simulink library "halin"  (R2021b)
settings: Solver=VariableStepAuto  StartTime=0.0  StopTime=10.0  RelTol=1e-3
undefined symbols (not defined in the file): TRUE
libraries: FVT_lib x177, hcu_lib x55
(part 6 of 17)

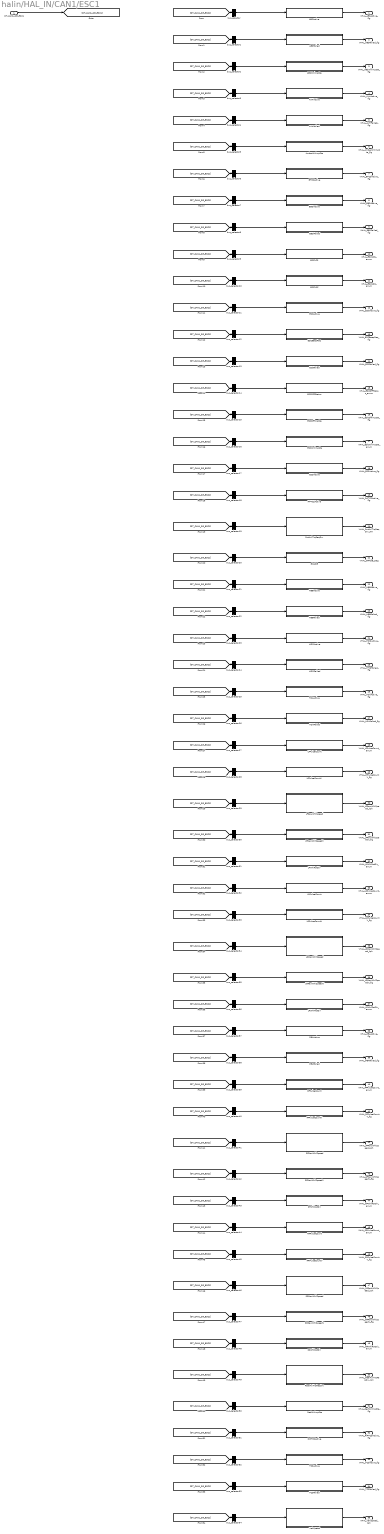
== system halin/HAL_IN/CAN1/ESC1 ==
  DT_CAN1_SG_ESC1 : Inport
  ABSActive : Subsystem
  ABSFailed : Subsystem
  ABSWnlmpSta : Subsystem
  AVHActive : Subsystem
  AVHFailed : Subsystem
  AmberWnlmpSta : Subsystem
  BTCSActive : Subsystem
  EBDActive : Subsystem
  EBDFailed : Subsystem
  ESC1CS : Subsystem
  ESC1RC : Subsystem
  ESCActive : Subsystem
  ESCBeepReq : Subsystem
  ESCFailed : Subsystem
  ESCOFFStatus : Subsystem
  ESCOfflmpSta : Subsystem
  ESCWnlmpSta : Subsystem
  ESSActive : Subsystem
  FrPTCSActive : Subsystem
  FrntAxlTrqReqDrv : Subsystem
  GRADE : Subsystem
  HBBActive : Subsystem
  HBBFailed : Subsystem
  HDDActive : Subsystem
  HDDFailed : Subsystem
  HSAActive : Subsystem
  HSAFailed : Subsystem
  LFPulseCount : Subsystem
  LFPulseCountV : Subsystem
  LFRawWhlSpeed : Subsystem
  LFRawWhlSpeedV : Subsystem
  LFWhlRotDir : Subsystem
  LRPulseCount : Subsystem
  LRPulseCountV : Subsystem
  LRRawWhlSpeed : Subsystem
  LRRawWhlSpeedV : Subsystem
  LRWhlRotDir : Subsystem
  PBAActive : Subsystem
  PBAFailed : Subsystem
  RFPulseCount : Subsystem
  RFPulseCountV : Subsystem
  RFRawWhlSpeed : Subsystem
  RFRawWhlSpeedV : Subsystem
  RFWhlRotDir : Subsystem
  RRPulseCount : Subsystem
  RRPulseCountV : Subsystem
  RRRawWhlSpeed : Subsystem
  RRRawWhlSpeedV : Subsystem
  RRWhlRotDir : Subsystem
  RearAxlTrqReqDrv : Subsystem
  RedWnlmpSta : Subsystem
  RrPTCSActive : Subsystem
  TCSActive : Subsystem
  TCSFailed : Subsystem
  VehSpeed : Subsystem
  bus_selector : BusSelector  OutputSignals=CAN1_ABS_Active
  bus_selector1 : BusSelector  OutputSignals=CAN1_ABS_Failed
  bus_selector10 : BusSelector  OutputSignals=CAN1_ESC1_RC
  bus_selector11 : BusSelector  OutputSignals=CAN1_ESC_Active
  bus_selector12 : BusSelector  OutputSignals=CAN1_ESC_BeepReq
  bus_selector13 : BusSelector  OutputSignals=CAN1_ESC_Failed
  bus_selector14 : BusSelector  OutputSignals=CAN1_ESC_OFF_Status
  bus_selector15 : BusSelector  OutputSignals=CAN1_ESC_Off_lmpSta
  bus_selector16 : BusSelector  OutputSignals=CAN1_ESC_WnlmpSta
  bus_selector17 : BusSelector  OutputSignals=CAN1_ESS_Active
  bus_selector18 : BusSelector  OutputSignals=CAN1_Fr_PTCS_Active
  bus_selector19 : BusSelector  OutputSignals=CAN1_FrntAxlTrqReq_Drv
  bus_selector2 : BusSelector  OutputSignals=CAN1_ABS_WnlmpSta
  bus_selector20 : BusSelector  OutputSignals=CAN1_GRADE
  bus_selector21 : BusSelector  OutputSignals=CAN1_HBB_Active
  bus_selector22 : BusSelector  OutputSignals=CAN1_HBB_Failed
  bus_selector23 : BusSelector  OutputSignals=CAN1_HDD_Active
  bus_selector24 : BusSelector  OutputSignals=CAN1_HDD_Failed
  bus_selector25 : BusSelector  OutputSignals=CAN1_HSA_Active
  bus_selector26 : BusSelector  OutputSignals=CAN1_HSA_Failed
  bus_selector27 : BusSelector  OutputSignals=CAN1_LF_PulseCount
  bus_selector28 : BusSelector  OutputSignals=CAN1_LF_PulseCount_V
  bus_selector29 : BusSelector  OutputSignals=CAN1_LF_RawWhlSpeed
  bus_selector3 : BusSelector  OutputSignals=CAN1_AVH_Active
  bus_selector30 : BusSelector  OutputSignals=CAN1_LF_RawWhlSpeed_V
  bus_selector31 : BusSelector  OutputSignals=CAN1_LF_WhlRotDir
  bus_selector32 : BusSelector  OutputSignals=CAN1_LR_PulseCount
  bus_selector33 : BusSelector  OutputSignals=CAN1_LR_PulseCount_V
  bus_selector34 : BusSelector  OutputSignals=CAN1_LR_RawWhlSpeed
  bus_selector35 : BusSelector  OutputSignals=CAN1_LR_RawWhlSpeed_V
  bus_selector36 : BusSelector  OutputSignals=CAN1_LR_WhlRotDir
  bus_selector37 : BusSelector  OutputSignals=CAN1_PBA_Active
  bus_selector38 : BusSelector  OutputSignals=CAN1_PBA_Failed
  bus_selector39 : BusSelector  OutputSignals=CAN1_RF_PulseCount
  bus_selector4 : BusSelector  OutputSignals=CAN1_AVH_Failed
  bus_selector40 : BusSelector  OutputSignals=CAN1_RF_PulseCount_V
  bus_selector41 : BusSelector  OutputSignals=CAN1_RF_RawWhlSpeed
  bus_selector42 : BusSelector  OutputSignals=CAN1_RF_RawWhlSpeed_V
  bus_selector43 : BusSelector  OutputSignals=CAN1_RF_WhlRotDir
  bus_selector44 : BusSelector  OutputSignals=CAN1_RR_PulseCount
  bus_selector45 : BusSelector  OutputSignals=CAN1_RR_PulseCount_V
  bus_selector46 : BusSelector  OutputSignals=CAN1_RR_RawWhlSpeed
  bus_selector47 : BusSelector  OutputSignals=CAN1_RR_RawWhlSpeed_V
  bus_selector48 : BusSelector  OutputSignals=CAN1_RR_WhlRotDir
  bus_selector49 : BusSelector  OutputSignals=CAN1_RearAxlTrqReq_Drv
  bus_selector5 : BusSelector  OutputSignals=CAN1_Amber_WnlmpSta
  bus_selector50 : BusSelector  OutputSignals=CAN1_Red_WnlmpSta
  bus_selector51 : BusSelector  OutputSignals=CAN1_Rr_PTCS_Active
  bus_selector52 : BusSelector  OutputSignals=CAN1_TCS_Active
  bus_selector53 : BusSelector  OutputSignals=CAN1_TCS_Failed
  bus_selector54 : BusSelector  OutputSignals=CAN1_VehSpeed
  bus_selector6 : BusSelector  OutputSignals=CAN1_BTCS_Active
  bus_selector7 : BusSelector  OutputSignals=CAN1_EBD_Active
  bus_selector8 : BusSelector  OutputSignals=CAN1_EBD_Failed
  bus_selector9 : BusSelector  OutputSignals=CAN1_ESC1_CS
  VHAL_ABSActive_flg : Outport
  VHAL_ABSFailed_flg : Outport  Port=2
  VHAL_ABSWnlmpSta_flg : Outport  Port=3
  VHAL_AVHActive_flg : Outport  Port=4
  VHAL_AVHFailed_flg : Outport  Port=5
  VHAL_AmberWnlmpSta_flg : Outport  Port=6
  VHAL_BTCSActive_flg : Outport  Port=7
  VHAL_EBDActive_flg : Outport  Port=8
  VHAL_EBDFailed_flg : Outport  Port=9
  VHAL_ESC1CS_enum : Outport  Port=10
  VHAL_ESC1RC_enum : Outport  Port=11
  VHAL_ESCActive_flg : Outport  Port=12
  VHAL_ESCBeepReq_flg : Outport  Port=13
  VHAL_ESCFailed_flg : Outport  Port=14
  VHAL_ESCOFFStatus_enum : Outport  Port=15
  VHAL_ESCOfflmpSta_flg : Outport  Port=16
  VHAL_ESCWnlmpSta_enum : Outport  Port=17
  VHAL_ESSActive_flg : Outport  Port=18
  VHAL_FrPTCSActive_flg : Outport  Port=19
  VHAL_FrntAxlTrqReqDrv_Nm : Outport  Port=20
  VHAL_GRADE_Deg : Outport  Port=21
  VHAL_HBBActive_flg : Outport  Port=22
  VHAL_HBBFailed_flg : Outport  Port=23
  VHAL_HDDActive_flg : Outport  Port=24
  VHAL_HDDFailed_flg : Outport  Port=25
  VHAL_HSAActive_flg : Outport  Port=26
  VHAL_HSAFailed_flg : Outport  Port=27
  VHAL_LFPulseCount_enum : Outport  Port=28
  VHAL_LFPulseCountV_flg : Outport  Port=29
  VHAL_LFRawWhlSpeed_kph : Outport  Port=30
  VHAL_LFRawWhlSpeedV_flg : Outport  Port=31
  VHAL_LFWhlRotDir_enum : Outport  Port=32
  VHAL_LRPulseCount_enum : Outport  Port=33
  VHAL_LRPulseCountV_flg : Outport  Port=34
  VHAL_LRRawWhlSpeed_kph : Outport  Port=35
  VHAL_LRRawWhlSpeedV_flg : Outport  Port=36
  VHAL_LRWhlRotDir_enum : Outport  Port=37
  VHAL_PBAActive_flg : Outport  Port=38
  VHAL_PBAFailed_flg : Outport  Port=39
  VHAL_RFPulseCount_enum : Outport  Port=40
  VHAL_RFPulseCountV_flg : Outport  Port=41
  VHAL_RFRawWhlSpeed_kph : Outport  Port=42
  VHAL_RFRawWhlSpeedV_flg : Outport  Port=43
  VHAL_RFWhlRotDir_enum : Outport  Port=44
  VHAL_RRPulseCount_enum : Outport  Port=45
  VHAL_RRPulseCountV_flg : Outport  Port=46
  VHAL_RRRawWhlSpeed_kph : Outport  Port=47
  VHAL_RRRawWhlSpeedV_flg : Outport  Port=48
  VHAL_RRWhlRotDir_enum : Outport  Port=49
  VHAL_RearAxlTrqReqDrv_Nm : Outport  Port=50
  VHAL_RedWnlmpSta_flg : Outport  Port=51
  VHAL_RrPTCSActive_flg : Outport  Port=52
  VHAL_TCSActive_flg : Outport  Port=53
  VHAL_TCSFailed_flg : Outport  Port=54
  VHAL_VehSpeed_kph : Outport  Port=55
  wires:
  DT_CAN1_SG_ESC1/1 -> [DT_CAN1_SG_ESC1]
  [DT_CAN1_SG_ESC1] -> bus_selector/1
  bus_selector/1 -> ABSActive/1(ABS_Active)  "<CAN1_ABS_Active>"
  ABSActive/1(VHAL_ABSActive_flg) -> VHAL_ABSActive_flg/1
  [DT_CAN1_SG_ESC1] -> bus_selector1/1
  bus_selector1/1 -> ABSFailed/1(ABS_Failed)  "<CAN1_ABS_Failed>"
  ABSFailed/1(VHAL_ABSFailed_flg) -> VHAL_ABSFailed_flg/1
  [DT_CAN1_SG_ESC1] -> bus_selector2/1
  bus_selector2/1 -> ABSWnlmpSta/1(ABS_WnlmpSta)  "<CAN1_ABS_WnlmpSta>"
  ABSWnlmpSta/1(VHAL_ABSWnlmpSta_flg) -> VHAL_ABSWnlmpSta_flg/1
  [DT_CAN1_SG_ESC1] -> bus_selector3/1
  bus_selector3/1 -> AVHActive/1(AVH_Active)  "<CAN1_AVH_Active>"
  AVHActive/1(VHAL_AVHActive_flg) -> VHAL_AVHActive_flg/1
  [DT_CAN1_SG_ESC1] -> bus_selector4/1
  bus_selector4/1 -> AVHFailed/1(AVH_Failed)  "<CAN1_AVH_Failed>"
  AVHFailed/1(VHAL_AVHFailed_flg) -> VHAL_AVHFailed_flg/1
  [DT_CAN1_SG_ESC1] -> bus_selector5/1
  bus_selector5/1 -> AmberWnlmpSta/1(Amber_WnlmpSta)  "<CAN1_Amber_WnlmpSta>"
  AmberWnlmpSta/1(VHAL_AmberWnlmpSta_flg) -> VHAL_AmberWnlmpSta_flg/1
  [DT_CAN1_SG_ESC1] -> bus_selector6/1
  bus_selector6/1 -> BTCSActive/1(BTCS_Active)  "<CAN1_BTCS_Active>"
  BTCSActive/1(VHAL_BTCSActive_flg) -> VHAL_BTCSActive_flg/1
  [DT_CAN1_SG_ESC1] -> bus_selector7/1
  bus_selector7/1 -> EBDActive/1(EBD_Active)  "<CAN1_EBD_Active>"
  EBDActive/1(VHAL_EBDActive_flg) -> VHAL_EBDActive_flg/1
  [DT_CAN1_SG_ESC1] -> bus_selector8/1
  bus_selector8/1 -> EBDFailed/1(EBD_Failed)  "<CAN1_EBD_Failed>"
  EBDFailed/1(VHAL_EBDFailed_flg) -> VHAL_EBDFailed_flg/1
  [DT_CAN1_SG_ESC1] -> bus_selector9/1
  bus_selector9/1 -> ESC1CS/1(ESC1_CS)  "<CAN1_ESC1_CS>"
  ESC1CS/1(VHAL_ESC1CS_enum) -> VHAL_ESC1CS_enum/1
  [DT_CAN1_SG_ESC1] -> bus_selector10/1
  bus_selector10/1 -> ESC1RC/1(ESC1_RC)  "<CAN1_ESC1_RC>"
  ESC1RC/1(VHAL_ESC1RC_enum) -> VHAL_ESC1RC_enum/1
  [DT_CAN1_SG_ESC1] -> bus_selector11/1
  bus_selector11/1 -> ESCActive/1(ESC_Active)  "<CAN1_ESC_Active>"
  ESCActive/1(VHAL_ESCActive_flg) -> VHAL_ESCActive_flg/1
  [DT_CAN1_SG_ESC1] -> bus_selector12/1
  bus_selector12/1 -> ESCBeepReq/1(ESC_BeepReq)  "<CAN1_ESC_BeepReq>"
  ESCBeepReq/1(VHAL_ESCBeepReq_flg) -> VHAL_ESCBeepReq_flg/1
  [DT_CAN1_SG_ESC1] -> bus_selector13/1
  bus_selector13/1 -> ESCFailed/1(ESC_Failed)  "<CAN1_ESC_Failed>"
  ESCFailed/1(VHAL_ESCFailed_flg) -> VHAL_ESCFailed_flg/1
  [DT_CAN1_SG_ESC1] -> bus_selector14/1
  bus_selector14/1 -> ESCOFFStatus/1(ESC_OFF_Status)  "<CAN1_ESC_OFF_Status>"
  ESCOFFStatus/1(VHAL_ESCOFFStatus_enum) -> VHAL_ESCOFFStatus_enum/1
  [DT_CAN1_SG_ESC1] -> bus_selector15/1
  bus_selector15/1 -> ESCOfflmpSta/1(ESC_Off_lmpSta)  "<CAN1_ESC_Off_lmpSta>"
  ESCOfflmpSta/1(VHAL_ESCOfflmpSta_flg) -> VHAL_ESCOfflmpSta_flg/1
  [DT_CAN1_SG_ESC1] -> bus_selector16/1
  bus_selector16/1 -> ESCWnlmpSta/1(ESC_WnlmpSta)  "<CAN1_ESC_WnlmpSta>"
  ESCWnlmpSta/1(VHAL_ESCWnlmpSta_enum) -> VHAL_ESCWnlmpSta_enum/1
  [DT_CAN1_SG_ESC1] -> bus_selector17/1
  bus_selector17/1 -> ESSActive/1(ESS_Active)  "<CAN1_ESS_Active>"
  ESSActive/1(VHAL_ESSActive_flg) -> VHAL_ESSActive_flg/1
  [DT_CAN1_SG_ESC1] -> bus_selector18/1
  bus_selector18/1 -> FrPTCSActive/1(Fr_PTCS_Active)  "<CAN1_Fr_PTCS_Active>"
  FrPTCSActive/1(VHAL_FrPTCSActive_flg) -> VHAL_FrPTCSActive_flg/1
  [DT_CAN1_SG_ESC1] -> bus_selector19/1
  bus_selector19/1 -> FrntAxlTrqReqDrv/1(FrntAxlTrqReq_Drv)  "<CAN1_FrntAxlTrqReq_Drv>"
  FrntAxlTrqReqDrv/1(VHAL_FrntAxlTrqReqDrv_Nm) -> VHAL_FrntAxlTrqReqDrv_Nm/1
  [DT_CAN1_SG_ESC1] -> bus_selector20/1
  bus_selector20/1 -> GRADE/1(GRADE)  "<CAN1_GRADE>"
  GRADE/1(VHAL_GRADE_Deg) -> VHAL_GRADE_Deg/1
  [DT_CAN1_SG_ESC1] -> bus_selector21/1
  bus_selector21/1 -> HBBActive/1(HBB_Active)  "<CAN1_HBB_Active>"
  HBBActive/1(VHAL_HBBActive_flg) -> VHAL_HBBActive_flg/1
  [DT_CAN1_SG_ESC1] -> bus_selector22/1
  bus_selector22/1 -> HBBFailed/1(HBB_Failed)  "<CAN1_HBB_Failed>"
  HBBFailed/1(VHAL_HBBFailed_flg) -> VHAL_HBBFailed_flg/1
  [DT_CAN1_SG_ESC1] -> bus_selector23/1
  bus_selector23/1 -> HDDActive/1(HDD_Active)  "<CAN1_HDD_Active>"
  HDDActive/1(VHAL_HDDActive_flg) -> VHAL_HDDActive_flg/1
  [DT_CAN1_SG_ESC1] -> bus_selector24/1
  bus_selector24/1 -> HDDFailed/1(HDD_Failed)  "<CAN1_HDD_Failed>"
  HDDFailed/1(VHAL_HDDFailed_flg) -> VHAL_HDDFailed_flg/1
  [DT_CAN1_SG_ESC1] -> bus_selector25/1
  bus_selector25/1 -> HSAActive/1(HSA_Active)  "<CAN1_HSA_Active>"
  HSAActive/1(VHAL_HSAActive_flg) -> VHAL_HSAActive_flg/1
  [DT_CAN1_SG_ESC1] -> bus_selector26/1
  bus_selector26/1 -> HSAFailed/1(HSA_Failed)  "<CAN1_HSA_Failed>"
  HSAFailed/1(VHAL_HSAFailed_flg) -> VHAL_HSAFailed_flg/1
  [DT_CAN1_SG_ESC1] -> bus_selector27/1
  bus_selector27/1 -> LFPulseCount/1(LF_PulseCount)  "<CAN1_LF_PulseCount>"
  LFPulseCount/1(VHAL_LFPulseCount_enum) -> VHAL_LFPulseCount_enum/1
  [DT_CAN1_SG_ESC1] -> bus_selector28/1
  bus_selector28/1 -> LFPulseCountV/1(LF_PulseCount_V)  "<CAN1_LF_PulseCount_V>"
  LFPulseCountV/1(VHAL_LFPulseCountV_flg) -> VHAL_LFPulseCountV_flg/1
  [DT_CAN1_SG_ESC1] -> bus_selector29/1
  bus_selector29/1 -> LFRawWhlSpeed/1(LF_RawWhlSpeed)  "<CAN1_LF_RawWhlSpeed>"
  LFRawWhlSpeed/1(VHAL_LFRawWhlSpeed_kph) -> VHAL_LFRawWhlSpeed_kph/1
  [DT_CAN1_SG_ESC1] -> bus_selector30/1
  bus_selector30/1 -> LFRawWhlSpeedV/1(LF_RawWhlSpeed_V)  "<CAN1_LF_RawWhlSpeed_V>"
  LFRawWhlSpeedV/1(VHAL_LFRawWhlSpeedV_flg) -> VHAL_LFRawWhlSpeedV_flg/1
  [DT_CAN1_SG_ESC1] -> bus_selector31/1
  bus_selector31/1 -> LFWhlRotDir/1(LF_WhlRotDir)  "<CAN1_LF_WhlRotDir>"
  LFWhlRotDir/1(VHAL_LFWhlRotDir_enum) -> VHAL_LFWhlRotDir_enum/1
  [DT_CAN1_SG_ESC1] -> bus_selector32/1
  bus_selector32/1 -> LRPulseCount/1(LR_PulseCount)  "<CAN1_LR_PulseCount>"
  LRPulseCount/1(VHAL_LRPulseCount_enum) -> VHAL_LRPulseCount_enum/1
  [DT_CAN1_SG_ESC1] -> bus_selector33/1
  bus_selector33/1 -> LRPulseCountV/1(LR_PulseCount_V)  "<CAN1_LR_PulseCount_V>"
  LRPulseCountV/1(VHAL_LRPulseCountV_flg) -> VHAL_LRPulseCountV_flg/1
  [DT_CAN1_SG_ESC1] -> bus_selector34/1
  bus_selector34/1 -> LRRawWhlSpeed/1(LR_RawWhlSpeed)  "<CAN1_LR_RawWhlSpeed>"
  LRRawWhlSpeed/1(VHAL_LRRawWhlSpeed_kph) -> VHAL_LRRawWhlSpeed_kph/1
  [DT_CAN1_SG_ESC1] -> bus_selector35/1
  bus_selector35/1 -> LRRawWhlSpeedV/1(LR_RawWhlSpeed_V)  "<CAN1_LR_RawWhlSpeed_V>"
  LRRawWhlSpeedV/1(VHAL_LRRawWhlSpeedV_flg) -> VHAL_LRRawWhlSpeedV_flg/1
  [DT_CAN1_SG_ESC1] -> bus_selector36/1
  bus_selector36/1 -> LRWhlRotDir/1(LR_WhlRotDir)  "<CAN1_LR_WhlRotDir>"
  LRWhlRotDir/1(VHAL_LRWhlRotDir_enum) -> VHAL_LRWhlRotDir_enum/1
  [DT_CAN1_SG_ESC1] -> bus_selector37/1
  bus_selector37/1 -> PBAActive/1(PBA_Active)  "<CAN1_PBA_Active>"
  PBAActive/1(VHAL_PBAActive_flg) -> VHAL_PBAActive_flg/1
  [DT_CAN1_SG_ESC1] -> bus_selector38/1
  bus_selector38/1 -> PBAFailed/1(PBA_Failed)  "<CAN1_PBA_Failed>"
  PBAFailed/1(VHAL_PBAFailed_flg) -> VHAL_PBAFailed_flg/1
  [DT_CAN1_SG_ESC1] -> bus_selector39/1
  bus_selector39/1 -> RFPulseCount/1(RF_PulseCount)  "<CAN1_RF_PulseCount>"
  RFPulseCount/1(VHAL_RFPulseCount_enum) -> VHAL_RFPulseCount_enum/1
  [DT_CAN1_SG_ESC1] -> bus_selector40/1
  bus_selector40/1 -> RFPulseCountV/1(RF_PulseCount_V)  "<CAN1_RF_PulseCount_V>"
  RFPulseCountV/1(VHAL_RFPulseCountV_flg) -> VHAL_RFPulseCountV_flg/1
  [DT_CAN1_SG_ESC1] -> bus_selector41/1
  bus_selector41/1 -> RFRawWhlSpeed/1(RF_RawWhlSpeed)  "<CAN1_RF_RawWhlSpeed>"
  RFRawWhlSpeed/1(VHAL_RFRawWhlSpeed_kph) -> VHAL_RFRawWhlSpeed_kph/1
  [DT_CAN1_SG_ESC1] -> bus_selector42/1
  bus_selector42/1 -> RFRawWhlSpeedV/1(RF_RawWhlSpeed_V)  "<CAN1_RF_RawWhlSpeed_V>"
  RFRawWhlSpeedV/1(VHAL_RFRawWhlSpeedV_flg) -> VHAL_RFRawWhlSpeedV_flg/1
  [DT_CAN1_SG_ESC1] -> bus_selector43/1
  bus_selector43/1 -> RFWhlRotDir/1(RF_WhlRotDir)  "<CAN1_RF_WhlRotDir>"
  RFWhlRotDir/1(VHAL_RFWhlRotDir_enum) -> VHAL_RFWhlRotDir_enum/1
  [DT_CAN1_SG_ESC1] -> bus_selector44/1
  bus_selector44/1 -> RRPulseCount/1(RR_PulseCount)  "<CAN1_RR_PulseCount>"
  RRPulseCount/1(VHAL_RRPulseCount_enum) -> VHAL_RRPulseCount_enum/1
  [DT_CAN1_SG_ESC1] -> bus_selector45/1
  bus_selector45/1 -> RRPulseCountV/1(RR_PulseCount_V)  "<CAN1_RR_PulseCount_V>"
  RRPulseCountV/1(VHAL_RRPulseCountV_flg) -> VHAL_RRPulseCountV_flg/1
  [DT_CAN1_SG_ESC1] -> bus_selector46/1
  bus_selector46/1 -> RRRawWhlSpeed/1(RR_RawWhlSpeed)  "<CAN1_RR_RawWhlSpeed>"
  RRRawWhlSpeed/1(VHAL_RRRawWhlSpeed_kph) -> VHAL_RRRawWhlSpeed_kph/1
  [DT_CAN1_SG_ESC1] -> bus_selector47/1
  bus_selector47/1 -> RRRawWhlSpeedV/1(RR_RawWhlSpeed_V)  "<CAN1_RR_RawWhlSpeed_V>"
  RRRawWhlSpeedV/1(VHAL_RRRawWhlSpeedV_flg) -> VHAL_RRRawWhlSpeedV_flg/1
  [DT_CAN1_SG_ESC1] -> bus_selector48/1
  bus_selector48/1 -> RRWhlRotDir/1(RR_WhlRotDir)  "<CAN1_RR_WhlRotDir>"
  RRWhlRotDir/1(VHAL_RRWhlRotDir_enum) -> VHAL_RRWhlRotDir_enum/1
  [DT_CAN1_SG_ESC1] -> bus_selector49/1
  bus_selector49/1 -> RearAxlTrqReqDrv/1(RearAxlTrqReq_Drv)  "<CAN1_RearAxlTrqReq_Drv>"
  RearAxlTrqReqDrv/1(VHAL_RearAxlTrqReqDrv_Nm) -> VHAL_RearAxlTrqReqDrv_Nm/1
  [DT_CAN1_SG_ESC1] -> bus_selector50/1
  bus_selector50/1 -> RedWnlmpSta/1(Red_WnlmpSta)  "<CAN1_Red_WnlmpSta>"
  RedWnlmpSta/1(VHAL_RedWnlmpSta_flg) -> VHAL_RedWnlmpSta_flg/1
  [DT_CAN1_SG_ESC1] -> bus_selector51/1
  bus_selector51/1 -> RrPTCSActive/1(Rr_PTCS_Active)  "<CAN1_Rr_PTCS_Active>"
  RrPTCSActive/1(VHAL_RrPTCSActive_flg) -> VHAL_RrPTCSActive_flg/1
  [DT_CAN1_SG_ESC1] -> bus_selector52/1
  bus_selector52/1 -> TCSActive/1(TCS_Active)  "<CAN1_TCS_Active>"
  TCSActive/1(VHAL_TCSActive_flg) -> VHAL_TCSActive_flg/1
  [DT_CAN1_SG_ESC1] -> bus_selector53/1
  bus_selector53/1 -> TCSFailed/1(TCS_Failed)  "<CAN1_TCS_Failed>"
  TCSFailed/1(VHAL_TCSFailed_flg) -> VHAL_TCSFailed_flg/1
  [DT_CAN1_SG_ESC1] -> bus_selector54/1
  bus_selector54/1 -> VehSpeed/1(VehSpeed)  "<CAN1_VehSpeed>"
  VehSpeed/1(VHAL_VehSpeed_kph) -> VHAL_VehSpeed_kph/1

== system halin/HAL_IN/CAN1/ESC5 ==
  DT_CAN1_SG_ESC5 : Inport
  ACCAvail : Subsystem
  AEBAvail : Subsystem
  ActBrkLampSta : Subsystem
  BrkDiscTempSta : Subsystem
  BrkPedalPos : Subsystem
  BrkPedalPosSta : Subsystem
  BrkSwSta : Subsystem
  BrkSwV : Subsystem
  ESC5CS : Subsystem
  ESC5RC : Subsystem
  ESCADASSta : Subsystem
  ESCAPSSta : Subsystem
  ESCStandstill : Subsystem
  FrRBCActive : Subsystem
  FrntAxlTrqReqBrk : Subsystem
  LatAccel : Subsystem
  LatAccelV : Subsystem
  LongAccel : Subsystem
  LongAccelV : Subsystem
  MCPressure : Subsystem
  MCPressureV : Subsystem
  MeterIndVehSpeed : Subsystem
  RDCActive : Subsystem
  RearAxlTrqReqBrk : Subsystem
  RrRBCActive : Subsystem
  YawRate : Subsystem
  YawRateV : Subsystem
  bus_selector : BusSelector  OutputSignals=CAN1_ACCAvail
  bus_selector1 : BusSelector  OutputSignals=CAN1_AEBAvail
  bus_selector10 : BusSelector  OutputSignals=CAN1_ESC_ADAS_Sta
  bus_selector11 : BusSelector  OutputSignals=CAN1_ESC_APS_Sta
  bus_selector12 : BusSelector  OutputSignals=CAN1_ESC_Standstill
  bus_selector13 : BusSelector  OutputSignals=CAN1_Fr_RBC_Active
  bus_selector14 : BusSelector  OutputSignals=CAN1_FrntAxlTrqReq_Brk
  bus_selector15 : BusSelector  OutputSignals=CAN1_LatAccel
  bus_selector16 : BusSelector  OutputSignals=CAN1_LatAccel_V
  bus_selector17 : BusSelector  OutputSignals=CAN1_LongAccel
  bus_selector18 : BusSelector  OutputSignals=CAN1_LongAccel_V
  bus_selector19 : BusSelector  OutputSignals=CAN1_MCPressure
  bus_selector2 : BusSelector  OutputSignals=CAN1_ActBrkLamp_Sta
  bus_selector20 : BusSelector  OutputSignals=CAN1_MCPressure_V
  bus_selector21 : BusSelector  OutputSignals=CAN1_Meter_Ind_VehSpeed
  bus_selector22 : BusSelector  OutputSignals=CAN1_RDC_Active
  bus_selector23 : BusSelector  OutputSignals=CAN1_RearAxlTrqReq_Brk
  bus_selector24 : BusSelector  OutputSignals=CAN1_Rr_RBC_Active
  bus_selector25 : BusSelector  OutputSignals=CAN1_YawRate
  bus_selector26 : BusSelector  OutputSignals=CAN1_YawRate_V
  bus_selector3 : BusSelector  OutputSignals=CAN1_BrkDiscTempSta
  bus_selector4 : BusSelector  OutputSignals=CAN1_BrkPedalPos
  bus_selector5 : BusSelector  OutputSignals=CAN1_BrkPedalPos_Sta
  bus_selector6 : BusSelector  OutputSignals=CAN1_BrkSw_Sta
  bus_selector7 : BusSelector  OutputSignals=CAN1_BrkSw_V
  bus_selector8 : BusSelector  OutputSignals=CAN1_ESC5_CS
  bus_selector9 : BusSelector  OutputSignals=CAN1_ESC5_RC
  VHAL_ACCAvail_flg : Outport
  VHAL_AEBAvail_flg : Outport  Port=2
  VHAL_ActBrkLampSta_flg : Outport  Port=3
  VHAL_BrkDiscTempSta_flg : Outport  Port=4
  VHAL_BrkPedalPos_pct : Outport  Port=5
  VHAL_BrkPedalPosSta_flg : Outport  Port=6
  VHAL_BrkSwSta_flg : Outport  Port=7
  VHAL_BrkSwV_flg : Outport  Port=8
  VHAL_ESC5CS_enum : Outport  Port=9
  VHAL_ESC5RC_enum : Outport  Port=10
  VHAL_ESCADASSta_enum : Outport  Port=11
  VHAL_ESCAPSSta_enum : Outport  Port=12
  VHAL_ESCStandstill_flg : Outport  Port=13
  VHAL_FrRBCActive_flg : Outport  Port=14
  VHAL_FrntAxlTrqReqBrk_Nm : Outport  Port=15
  VHAL_LatAccel_Gps : Outport  Port=16
  VHAL_LatAccelV_flg : Outport  Port=17
  VHAL_LongAccel_Gps : Outport  Port=18
  VHAL_LongAccelV_flg : Outport  Port=19
  VHAL_MCPressure_bar : Outport  Port=20
  VHAL_MCPressureV_flg : Outport  Port=21
  VHAL_MeterIndVehSpeed_kph : Outport  Port=22
  VHAL_RDCActive_enum : Outport  Port=23
  VHAL_RearAxlTrqReqBrk_Nm : Outport  Port=24
  VHAL_RrRBCActive_flg : Outport  Port=25
  VHAL_YawRate_degps : Outport  Port=26
  VHAL_YawRateV_flg : Outport  Port=27
  wires:
  DT_CAN1_SG_ESC5/1 -> [DT_CAN1_SG_ESC5]
  [DT_CAN1_SG_ESC5] -> bus_selector/1
  bus_selector/1 -> ACCAvail/1(ACCAvail)  "<CAN1_ACCAvail>"
  ACCAvail/1(VHAL_ACCAvail_flg) -> VHAL_ACCAvail_flg/1
  [DT_CAN1_SG_ESC5] -> bus_selector1/1
  bus_selector1/1 -> AEBAvail/1(AEBAvail)  "<CAN1_AEBAvail>"
  AEBAvail/1(VHAL_AEBAvail_flg) -> VHAL_AEBAvail_flg/1
  [DT_CAN1_SG_ESC5] -> bus_selector2/1
  bus_selector2/1 -> ActBrkLampSta/1(ActBrkLamp_Sta)  "<CAN1_ActBrkLamp_Sta>"
  ActBrkLampSta/1(VHAL_ActBrkLampSta_flg) -> VHAL_ActBrkLampSta_flg/1
  [DT_CAN1_SG_ESC5] -> bus_selector3/1
  bus_selector3/1 -> BrkDiscTempSta/1(BrkDiscTempSta)  "<CAN1_BrkDiscTempSta>"
  BrkDiscTempSta/1(VHAL_BrkDiscTempSta_flg) -> VHAL_BrkDiscTempSta_flg/1
  [DT_CAN1_SG_ESC5] -> bus_selector4/1
  bus_selector4/1 -> BrkPedalPos/1(BrkPedalPos)  "<CAN1_BrkPedalPos>"
  BrkPedalPos/1(VHAL_BrkPedalPos_pct) -> VHAL_BrkPedalPos_pct/1
  [DT_CAN1_SG_ESC5] -> bus_selector5/1
  bus_selector5/1 -> BrkPedalPosSta/1(BrkPedalPos_Sta)  "<CAN1_BrkPedalPos_Sta>"
  BrkPedalPosSta/1(VHAL_BrkPedalPosSta_flg) -> VHAL_BrkPedalPosSta_flg/1
  [DT_CAN1_SG_ESC5] -> bus_selector6/1
  bus_selector6/1 -> BrkSwSta/1(BrkSw_Sta)  "<CAN1_BrkSw_Sta>"
  BrkSwSta/1(VHAL_BrkSwSta_flg) -> VHAL_BrkSwSta_flg/1
  [DT_CAN1_SG_ESC5] -> bus_selector7/1
  bus_selector7/1 -> BrkSwV/1(BrkSw_V)  "<CAN1_BrkSw_V>"
  BrkSwV/1(VHAL_BrkSwV_flg) -> VHAL_BrkSwV_flg/1
  [DT_CAN1_SG_ESC5] -> bus_selector8/1
  bus_selector8/1 -> ESC5CS/1(ESC5_CS)  "<CAN1_ESC5_CS>"
  ESC5CS/1(VHAL_ESC5CS_enum) -> VHAL_ESC5CS_enum/1
  [DT_CAN1_SG_ESC5] -> bus_selector9/1
  bus_selector9/1 -> ESC5RC/1(ESC5_RC)  "<CAN1_ESC5_RC>"
  ESC5RC/1(VHAL_ESC5RC_enum) -> VHAL_ESC5RC_enum/1
  [DT_CAN1_SG_ESC5] -> bus_selector10/1
  bus_selector10/1 -> ESCADASSta/1(ESC_ADAS_Sta)  "<CAN1_ESC_ADAS_Sta>"
  ESCADASSta/1(VHAL_ESCADASSta_enum) -> VHAL_ESCADASSta_enum/1
  [DT_CAN1_SG_ESC5] -> bus_selector11/1
  bus_selector11/1 -> ESCAPSSta/1(ESC_APS_Sta)  "<CAN1_ESC_APS_Sta>"
  ESCAPSSta/1(VHAL_ESCAPSSta_enum) -> VHAL_ESCAPSSta_enum/1
  [DT_CAN1_SG_ESC5] -> bus_selector12/1
  bus_selector12/1 -> ESCStandstill/1(ESC_Standstill)  "<CAN1_ESC_Standstill>"
  ESCStandstill/1(VHAL_ESCStandstill_flg) -> VHAL_ESCStandstill_flg/1
  [DT_CAN1_SG_ESC5] -> bus_selector13/1
  bus_selector13/1 -> FrRBCActive/1(Fr_RBC_Active)  "<CAN1_Fr_RBC_Active>"
  FrRBCActive/1(VHAL_FrRBCActive_flg) -> VHAL_FrRBCActive_flg/1
  [DT_CAN1_SG_ESC5] -> bus_selector14/1
  bus_selector14/1 -> FrntAxlTrqReqBrk/1(FrntAxlTrqReq_Brk)  "<CAN1_FrntAxlTrqReq_Brk>"
  FrntAxlTrqReqBrk/1(VHAL_FrntAxlTrqReqBrk_Nm) -> VHAL_FrntAxlTrqReqBrk_Nm/1
  [DT_CAN1_SG_ESC5] -> bus_selector15/1
  bus_selector15/1 -> LatAccel/1(LatAccel)  "<CAN1_LatAccel>"
  LatAccel/1(VHAL_LatAccel_Gps) -> VHAL_LatAccel_Gps/1
  [DT_CAN1_SG_ESC5] -> bus_selector16/1
  bus_selector16/1 -> LatAccelV/1(LatAccel_V)  "<CAN1_LatAccel_V>"
  LatAccelV/1(VHAL_LatAccelV_flg) -> VHAL_LatAccelV_flg/1
  [DT_CAN1_SG_ESC5] -> bus_selector17/1
  bus_selector17/1 -> LongAccel/1(LongAccel)  "<CAN1_LongAccel>"
  LongAccel/1(VHAL_LongAccel_Gps) -> VHAL_LongAccel_Gps/1
  [DT_CAN1_SG_ESC5] -> bus_selector18/1
  bus_selector18/1 -> LongAccelV/1(LongAccel_V)  "<CAN1_LongAccel_V>"
  LongAccelV/1(VHAL_LongAccelV_flg) -> VHAL_LongAccelV_flg/1
  [DT_CAN1_SG_ESC5] -> bus_selector19/1
  bus_selector19/1 -> MCPressure/1(MCPressure)  "<CAN1_MCPressure>"
  MCPressure/1(VHAL_MCPressure_bar) -> VHAL_MCPressure_bar/1
  [DT_CAN1_SG_ESC5] -> bus_selector20/1
  bus_selector20/1 -> MCPressureV/1(MCPressure_V)  "<CAN1_MCPressure_V>"
  MCPressureV/1(VHAL_MCPressureV_flg) -> VHAL_MCPressureV_flg/1
  [DT_CAN1_SG_ESC5] -> bus_selector21/1
  bus_selector21/1 -> MeterIndVehSpeed/1(Meter_Ind_VehSpeed)  "<CAN1_Meter_Ind_VehSpeed>"
  MeterIndVehSpeed/1(VHAL_MeterIndVehSpeed_kph) -> VHAL_MeterIndVehSpeed_kph/1
  [DT_CAN1_SG_ESC5] -> bus_selector22/1
  bus_selector22/1 -> RDCActive/1(RDC_Active)  "<CAN1_RDC_Active>"
  RDCActive/1(VHAL_RDCActive_enum) -> VHAL_RDCActive_enum/1
  [DT_CAN1_SG_ESC5] -> bus_selector23/1
  bus_selector23/1 -> RearAxlTrqReqBrk/1(RearAxlTrqReq_Brk)  "<CAN1_RearAxlTrqReq_Brk>"
  RearAxlTrqReqBrk/1(VHAL_RearAxlTrqReqBrk_Nm) -> VHAL_RearAxlTrqReqBrk_Nm/1
  [DT_CAN1_SG_ESC5] -> bus_selector24/1
  bus_selector24/1 -> RrRBCActive/1(Rr_RBC_Active)  "<CAN1_Rr_RBC_Active>"
  RrRBCActive/1(VHAL_RrRBCActive_flg) -> VHAL_RrRBCActive_flg/1
  [DT_CAN1_SG_ESC5] -> bus_selector25/1
  bus_selector25/1 -> YawRate/1(YawRate)  "<CAN1_YawRate>"
  YawRate/1(VHAL_YawRate_degps) -> VHAL_YawRate_degps/1
  [DT_CAN1_SG_ESC5] -> bus_selector26/1
  bus_selector26/1 -> YawRateV/1(YawRate_V)  "<CAN1_YawRate_V>"
  YawRateV/1(VHAL_YawRateV_flg) -> VHAL_YawRateV_flg/1

== system halin/HAL_IN/CAN1/VHAL_CANMsgInvalidABM1_flg ==
  Cast To Boolean13 : DataTypeConversion  OutDataTypeStr=boolean
  Constant : Constant  Value=TRUE
  Latch13 : hcu_lib/Basic_Blocks/Latch
  Switch13 : Switch  Criteria=u2 ~= 0
  Unit Delay : UnitDelay  SampleTime=-1  HasFrameUpgradeWarning=on
  UnitConverter : DataTypeConversion  OutDataTypeStr=boolean
  Out : Outport
  wires:
  Constant/1 -> Switch13/3
  Unit Delay/1 -> Cast To Boolean13/1
  Cast To Boolean13/1 -> Switch13/1, Latch13/1
  Switch13/1 -> UnitConverter/1
  Latch13/1 -> Switch13/2
  UnitConverter/1 -> Unit Delay/1, Out/1  "VHAL_CANMsgInvalidABM1_flg"

== system halin/HAL_IN/CAN1/VHAL_CANMsgInvalidEPB1_flg ==
  Cast To Boolean13 : DataTypeConversion  OutDataTypeStr=boolean
  Constant : Constant  Value=TRUE
  Latch13 : hcu_lib/Basic_Blocks/Latch
  Switch13 : Switch  Criteria=u2 ~= 0
  Unit Delay : UnitDelay  SampleTime=-1  HasFrameUpgradeWarning=on
  UnitConverter : DataTypeConversion  OutDataTypeStr=boolean
  Out : Outport
  wires:
  Constant/1 -> Switch13/3
  Unit Delay/1 -> Cast To Boolean13/1
  Cast To Boolean13/1 -> Switch13/1, Latch13/1
  Switch13/1 -> UnitConverter/1
  Latch13/1 -> Switch13/2
  UnitConverter/1 -> Unit Delay/1, Out/1  "VHAL_CANMsgInvalidEPB1_flg"

== system halin/HAL_IN/CAN1/VHAL_CANMsgInvalidEPS1_flg ==
  Cast To Boolean13 : DataTypeConversion  OutDataTypeStr=boolean
  Constant : Constant  Value=TRUE
  Latch13 : hcu_lib/Basic_Blocks/Latch
  Switch13 : Switch  Criteria=u2 ~= 0
  Unit Delay : UnitDelay  SampleTime=-1  HasFrameUpgradeWarning=on
  UnitConverter : DataTypeConversion  OutDataTypeStr=boolean
  Out : Outport
  wires:
  Constant/1 -> Switch13/3
  Unit Delay/1 -> Cast To Boolean13/1
  Cast To Boolean13/1 -> Switch13/1, Latch13/1
  Switch13/1 -> UnitConverter/1
  Latch13/1 -> Switch13/2
  UnitConverter/1 -> Unit Delay/1, Out/1  "VHAL_CANMsgInvalidEPS1_flg"

== system halin/HAL_IN/CAN1/VHAL_CANMsgInvalidESC1_flg ==
  Cast To Boolean13 : DataTypeConversion  OutDataTypeStr=boolean
  Constant : Constant  Value=TRUE
  Latch13 : hcu_lib/Basic_Blocks/Latch
  Switch13 : Switch  Criteria=u2 ~= 0
  Unit Delay : UnitDelay  SampleTime=-1  HasFrameUpgradeWarning=on
  UnitConverter : DataTypeConversion  OutDataTypeStr=boolean
  Out : Outport
  wires:
  Constant/1 -> Switch13/3
  Unit Delay/1 -> Cast To Boolean13/1
  Cast To Boolean13/1 -> Switch13/1, Latch13/1
  Switch13/1 -> UnitConverter/1
  Latch13/1 -> Switch13/2
  UnitConverter/1 -> Unit Delay/1, Out/1  "VHAL_CANMsgInvalidESC1_flg"

== system halin/HAL_IN/CAN1/VHAL_CANMsgInvalidESC5_flg ==
  Cast To Boolean13 : DataTypeConversion  OutDataTypeStr=boolean
  Constant : Constant  Value=TRUE
  Latch13 : hcu_lib/Basic_Blocks/Latch
  Switch13 : Switch  Criteria=u2 ~= 0
  Unit Delay : UnitDelay  SampleTime=-1  HasFrameUpgradeWarning=on
  UnitConverter : DataTypeConversion  OutDataTypeStr=boolean
  Out : Outport
  wires:
  Constant/1 -> Switch13/3
  Unit Delay/1 -> Cast To Boolean13/1
  Cast To Boolean13/1 -> Switch13/1, Latch13/1
  Switch13/1 -> UnitConverter/1
  Latch13/1 -> Switch13/2
  UnitConverter/1 -> Unit Delay/1, Out/1  "VHAL_CANMsgInvalidESC5_flg"

== system halin/HAL_IN/CAN1/VHAL_CANMsgInvalideBST1_flg ==
  Cast To Boolean13 : DataTypeConversion  OutDataTypeStr=boolean
  Constant : Constant  Value=TRUE
  Latch13 : hcu_lib/Basic_Blocks/Latch
  Switch13 : Switch  Criteria=u2 ~= 0
  Unit Delay : UnitDelay  SampleTime=-1  HasFrameUpgradeWarning=on
  UnitConverter : DataTypeConversion  OutDataTypeStr=boolean
  Out : Outport
  wires:
  Constant/1 -> Switch13/3
  Unit Delay/1 -> Cast To Boolean13/1
  Cast To Boolean13/1 -> Switch13/1, Latch13/1
  Switch13/1 -> UnitConverter/1
  Latch13/1 -> Switch13/2
  UnitConverter/1 -> Unit Delay/1, Out/1  "VHAL_CANMsgInvalideBST1_flg"

== system halin/HAL_IN/CAN1/eBST1 ==
  DT_CAN1_SG_eBST1 : Inport
  LowBrakeFluidSta : Subsystem
  bus_selector : BusSelector  OutputSignals=CAN1_LowBrakeFluid_Sta
  bus_selector1 : BusSelector  OutputSignals=CAN1_eBST_AmberWnlmpSta
  bus_selector2 : BusSelector  OutputSignals=CAN1_eBST_BeepReq
  bus_selector3 : BusSelector  OutputSignals=CAN1_eBST_RedWnlmpSta
  eBSTAmberWnlmpSta : Subsystem
  eBSTBeepReq : Subsystem
  eBSTRedWnlmpSta : Subsystem
  VHAL_LowBrakeFluidSta_flg : Outport
  VHAL_eBSTAmberWnlmpSta_flg : Outport  Port=2
  VHAL_eBSTBeepReq_flg : Outport  Port=3
  VHAL_eBSTRedWnlmpSta_flg : Outport  Port=4
  wires:
  DT_CAN1_SG_eBST1/1 -> [DT_CAN1_SG_eBST1]
  [DT_CAN1_SG_eBST1] -> bus_selector/1
  bus_selector/1 -> LowBrakeFluidSta/1(LowBrakeFluid_Sta)  "<CAN1_LowBrakeFluid_Sta>"
  LowBrakeFluidSta/1(VHAL_LowBrakeFluidSta_flg) -> VHAL_LowBrakeFluidSta_flg/1
  [DT_CAN1_SG_eBST1] -> bus_selector1/1
  bus_selector1/1 -> eBSTAmberWnlmpSta/1(eBST_AmberWnlmpSta)  "<CAN1_eBST_AmberWnlmpSta>"
  eBSTAmberWnlmpSta/1(VHAL_eBSTAmberWnlmpSta_flg) -> VHAL_eBSTAmberWnlmpSta_flg/1
  [DT_CAN1_SG_eBST1] -> bus_selector2/1
  bus_selector2/1 -> eBSTBeepReq/1(eBST_BeepReq)  "<CAN1_eBST_BeepReq>"
  eBSTBeepReq/1(VHAL_eBSTBeepReq_flg) -> VHAL_eBSTBeepReq_flg/1
  [DT_CAN1_SG_eBST1] -> bus_selector3/1
  bus_selector3/1 -> eBSTRedWnlmpSta/1(eBST_RedWnlmpSta)  "<CAN1_eBST_RedWnlmpSta>"
  eBSTRedWnlmpSta/1(VHAL_eBSTRedWnlmpSta_flg) -> VHAL_eBSTRedWnlmpSta_flg/1

== system halin/HAL_IN/CAN2/HMI1 ==
  DT_CAN2_SG_HMI1 : Inport
  HMIACAirIntMCmd : Subsystem
  HMIACAirIntPCmd : Subsystem
  HMIACAutoBtnCmd : Subsystem
  HMIACBtnCmd : Subsystem
  HMIACFrDefogBtnCmd : Subsystem
  HMIACRecycleBtnCmd : Subsystem
  HMIACWindDirMCmd : Subsystem
  HMIACWindDirPCmd : Subsystem
  HMIZ1SetTMCmd : Subsystem
  HMIZ1SetTPCmd : Subsystem
  HMIZ2SetTMCmd : Subsystem
  HMIZ2SetTPCmd : Subsystem
  bus_selector : BusSelector  OutputSignals=CAN2_HMI_ACAirIntM_Cmd
  bus_selector1 : BusSelector  OutputSignals=CAN2_HMI_ACAirIntP_Cmd
  bus_selector10 : BusSelector  OutputSignals=CAN2_HMI_Z2SetTM_Cmd
  bus_selector11 : BusSelector  OutputSignals=CAN2_HMI_Z2SetTP_Cmd
  bus_selector2 : BusSelector  OutputSignals=CAN2_HMI_ACAutoBtn_Cmd
  bus_selector3 : BusSelector  OutputSignals=CAN2_HMI_ACBtn_Cmd
  bus_selector4 : BusSelector  OutputSignals=CAN2_HMI_ACFrDefogBtn_Cmd
  bus_selector5 : BusSelector  OutputSignals=CAN2_HMI_ACRecycleBtn_Cmd
  bus_selector6 : BusSelector  OutputSignals=CAN2_HMI_ACWindDirM_Cmd
  bus_selector7 : BusSelector  OutputSignals=CAN2_HMI_ACWindDirP_Cmd
  bus_selector8 : BusSelector  OutputSignals=CAN2_HMI_Z1SetTM_Cmd
  bus_selector9 : BusSelector  OutputSignals=CAN2_HMI_Z1SetTP_Cmd
  VHAL_HMIACAirIntMCmd_flg : Outport
  VHAL_HMIACAirIntPCmd_flg : Outport  Port=2
  VHAL_HMIACAutoBtnCmd_flg : Outport  Port=3
  VHAL_HMIACBtnCmd_flg : Outport  Port=4
  VHAL_HMIACFrDefogBtnCmd_flg : Outport  Port=5
  VHAL_HMIACRecycleBtnCmd_flg : Outport  Port=6
  VHAL_HMIACWindDirMCmd_flg : Outport  Port=7
  VHAL_HMIACWindDirPCmd_flg : Outport  Port=8
  VHAL_HMIZ1SetTMCmd_flg : Outport  Port=9
  VHAL_HMIZ1SetTPCmd_flg : Outport  Port=10
  VHAL_HMIZ2SetTMCmd_flg : Outport  Port=11
  VHAL_HMIZ2SetTPCmd_flg : Outport  Port=12
  wires:
  DT_CAN2_SG_HMI1/1 -> [DT_CAN2_SG_HMI1]
  [DT_CAN2_SG_HMI1] -> bus_selector/1
  bus_selector/1 -> HMIACAirIntMCmd/1(HMI_ACAirIntM_Cmd)  "<CAN2_HMI_ACAirIntM_Cmd>"
  HMIACAirIntMCmd/1(VHAL_HMIACAirIntMCmd_flg) -> VHAL_HMIACAirIntMCmd_flg/1
  [DT_CAN2_SG_HMI1] -> bus_selector1/1
  bus_selector1/1 -> HMIACAirIntPCmd/1(HMI_ACAirIntP_Cmd)  "<CAN2_HMI_ACAirIntP_Cmd>"
  HMIACAirIntPCmd/1(VHAL_HMIACAirIntPCmd_flg) -> VHAL_HMIACAirIntPCmd_flg/1
  [DT_CAN2_SG_HMI1] -> bus_selector2/1
  bus_selector2/1 -> HMIACAutoBtnCmd/1(HMI_ACAutoBtn_Cmd)  "<CAN2_HMI_ACAutoBtn_Cmd>"
  HMIACAutoBtnCmd/1(VHAL_HMIACAutoBtnCmd_flg) -> VHAL_HMIACAutoBtnCmd_flg/1
  [DT_CAN2_SG_HMI1] -> bus_selector3/1
  bus_selector3/1 -> HMIACBtnCmd/1(HMI_ACBtn_Cmd)  "<CAN2_HMI_ACBtn_Cmd>"
  HMIACBtnCmd/1(VHAL_HMIACBtnCmd_flg) -> VHAL_HMIACBtnCmd_flg/1
  [DT_CAN2_SG_HMI1] -> bus_selector4/1
  bus_selector4/1 -> HMIACFrDefogBtnCmd/1(HMI_ACFrDefogBtn_Cmd)  "<CAN2_HMI_ACFrDefogBtn_Cmd>"
  HMIACFrDefogBtnCmd/1(VHAL_HMIACFrDefogBtnCmd_flg) -> VHAL_HMIACFrDefogBtnCmd_flg/1
  [DT_CAN2_SG_HMI1] -> bus_selector5/1
  bus_selector5/1 -> HMIACRecycleBtnCmd/1(HMI_ACRecycleBtn_Cmd)  "<CAN2_HMI_ACRecycleBtn_Cmd>"
  HMIACRecycleBtnCmd/1(VHAL_HMIACRecycleBtnCmd_flg) -> VHAL_HMIACRecycleBtnCmd_flg/1
  [DT_CAN2_SG_HMI1] -> bus_selector6/1
  bus_selector6/1 -> HMIACWindDirMCmd/1(HMI_ACWindDirM_Cmd)  "<CAN2_HMI_ACWindDirM_Cmd>"
  HMIACWindDirMCmd/1(VHAL_HMIACWindDirMCmd_flg) -> VHAL_HMIACWindDirMCmd_flg/1
  [DT_CAN2_SG_HMI1] -> bus_selector7/1
  bus_selector7/1 -> HMIACWindDirPCmd/1(HMI_ACWindDirP_Cmd)  "<CAN2_HMI_ACWindDirP_Cmd>"
  HMIACWindDirPCmd/1(VHAL_HMIACWindDirPCmd_flg) -> VHAL_HMIACWindDirPCmd_flg/1
  [DT_CAN2_SG_HMI1] -> bus_selector8/1
  bus_selector8/1 -> HMIZ1SetTMCmd/1(HMI_Z1SetTM_Cmd)  "<CAN2_HMI_Z1SetTM_Cmd>"
  HMIZ1SetTMCmd/1(VHAL_HMIZ1SetTMCmd_flg) -> VHAL_HMIZ1SetTMCmd_flg/1
  [DT_CAN2_SG_HMI1] -> bus_selector9/1
  bus_selector9/1 -> HMIZ1SetTPCmd/1(HMI_Z1SetTP_Cmd)  "<CAN2_HMI_Z1SetTP_Cmd>"
  HMIZ1SetTPCmd/1(VHAL_HMIZ1SetTPCmd_flg) -> VHAL_HMIZ1SetTPCmd_flg/1
  [DT_CAN2_SG_HMI1] -> bus_selector10/1
  bus_selector10/1 -> HMIZ2SetTMCmd/1(HMI_Z2SetTM_Cmd)  "<CAN2_HMI_Z2SetTM_Cmd>"
  HMIZ2SetTMCmd/1(VHAL_HMIZ2SetTMCmd_flg) -> VHAL_HMIZ2SetTMCmd_flg/1
  [DT_CAN2_SG_HMI1] -> bus_selector11/1
  bus_selector11/1 -> HMIZ2SetTPCmd/1(HMI_Z2SetTP_Cmd)  "<CAN2_HMI_Z2SetTP_Cmd>"
  HMIZ2SetTPCmd/1(VHAL_HMIZ2SetTPCmd_flg) -> VHAL_HMIZ2SetTPCmd_flg/1

== system halin/HAL_IN/CAN2/IVI1 ==
  DT_CAN2_SG_IVI1 : Inport
  AmbLighLowBatAlertSW : Subsystem
  AmbLighSafetyAlertSW : Subsystem
  AmbLightBrightnessSet : Subsystem
  AmbLightColorSet : Subsystem
  AmbLightDimInDarkSW : Subsystem
  AmbLightSW : Subsystem
  AmbLightWlcmLightSW : Subsystem
  FCPFrEvtBtnACMaxReq : Subsystem
  FCPFrEvtBtnACReq : Subsystem
  FCPFrEvtBtnAutoReq : Subsystem
  FCPFrEvtBtnSyncReq : Subsystem
  IVICreateAccReqSta : Subsystem
  IVIDelAccReqSta : Subsystem
  IVILinkAccReqSta : Subsystem
  IVILinkAccSta : Subsystem
  IVILinkKeySta : Subsystem
  IVILocatedSTA : Subsystem
  IVILockSoundSWSta : Subsystem
  IVITimeCheck : Subsystem
  IVITimeDay : Subsystem
  IVITimeHour : Subsystem
  IVITimeMinute : Subsystem
  IVITimeMonth : Subsystem
  IVITimeSecond : Subsystem
  IVITimeYear : Subsystem
  LINKtoDrive : Subsystem
  OpenDrOpenWdoSW : Subsystem
  PWCONTINUEUSE : Subsystem
  SmartEcoModeSW : Subsystem
  UserSet : Subsystem
  bus_selector : BusSelector  OutputSignals=CAN2_AmbLigh_LowBatAlert_SW
  bus_selector1 : BusSelector  OutputSignals=CAN2_AmbLigh_SafetyAlert_SW
  bus_selector10 : BusSelector  OutputSignals=CAN2_FCP_FrEvt_BtnSyncReq
  bus_selector11 : BusSelector  OutputSignals=CAN2_IVI_CreateAccReq_Sta
  bus_selector12 : BusSelector  OutputSignals=CAN2_IVI_DelAccReq_Sta
  bus_selector13 : BusSelector  OutputSignals=CAN2_IVI_LinkAccReq_Sta
  bus_selector14 : BusSelector  OutputSignals=CAN2_IVI_LinkAcc_Sta
  bus_selector15 : BusSelector  OutputSignals=CAN2_IVI_LinkKey_Sta
  bus_selector16 : BusSelector  OutputSignals=CAN2_IVI_Located_STA
  bus_selector17 : BusSelector  OutputSignals=CAN2_IVI_Lock_SoundSW_Sta
  bus_selector18 : BusSelector  OutputSignals=CAN2_IVI_Time_Check
  bus_selector19 : BusSelector  OutputSignals=CAN2_IVI_Time_Day
  bus_selector2 : BusSelector  OutputSignals=CAN2_AmbLightBrightnessSet
  bus_selector20 : BusSelector  OutputSignals=CAN2_IVI_Time_Hour
  bus_selector21 : BusSelector  OutputSignals=CAN2_IVI_Time_Minute
  bus_selector22 : BusSelector  OutputSignals=CAN2_IVI_Time_Month
  bus_selector23 : BusSelector  OutputSignals=CAN2_IVI_Time_Second
  bus_selector24 : BusSelector  OutputSignals=CAN2_IVI_Time_Year
  bus_selector25 : BusSelector  OutputSignals=CAN2_LINKtoDrive
  bus_selector26 : BusSelector  OutputSignals=CAN2_OpenDrOpenWdo_SW
  bus_selector27 : BusSelector  OutputSignals=CAN2_PW_CONTINUE_USE
  bus_selector28 : BusSelector  OutputSignals=CAN2_SmartEco_Mode_SW
  bus_selector29 : BusSelector  OutputSignals=CAN2_UserSet
  bus_selector3 : BusSelector  OutputSignals=CAN2_AmbLightColorSet
  bus_selector4 : BusSelector  OutputSignals=CAN2_AmbLight_DimInDark_SW
  bus_selector5 : BusSelector  OutputSignals=CAN2_AmbLight_SW
  bus_selector6 : BusSelector  OutputSignals=CAN2_AmbLight_WlcmLight_SW
  bus_selector7 : BusSelector  OutputSignals=CAN2_FCP_FrEvt_BtnACMaxReq
  bus_selector8 : BusSelector  OutputSignals=CAN2_FCP_FrEvt_BtnACReq
  bus_selector9 : BusSelector  OutputSignals=CAN2_FCP_FrEvt_BtnAutoReq
  VHAL_AmbLighLowBatAlertSW_flg : Outport
  VHAL_AmbLighSafetyAlertSW_flg : Outport  Port=2
  VHAL_AmbLightBrightnessSet_enum : Outport  Port=3
  VHAL_AmbLightColorSet_enum : Outport  Port=4
  VHAL_AmbLightDimInDarkSW_flg : Outport  Port=5
  VHAL_AmbLightSW_flg : Outport  Port=6
  VHAL_AmbLightWlcmLightSW_flg : Outport  Port=7
  VHAL_FCPFrEvtBtnACMaxReq_flg : Outport  Port=8
  VHAL_FCPFrEvtBtnACReq_flg : Outport  Port=9
  VHAL_FCPFrEvtBtnAutoReq_flg : Outport  Port=10
  VHAL_FCPFrEvtBtnSyncReq_flg : Outport  Port=11
  VHAL_IVICreateAccReqSta_enum : Outport  Port=12
  VHAL_IVIDelAccReqSta_enum : Outport  Port=13
  VHAL_IVILinkAccReqSta_flg : Outport  Port=14
  VHAL_IVILinkAccSta_enum : Outport  Port=15
  VHAL_IVILinkKeySta_enum : Outport  Port=16
  VHAL_IVILocatedSTA_enum : Outport  Port=17
  VHAL_IVILockSoundSWSta_flg : Outport  Port=18
  VHAL_IVITimeCheck_enum : Outport  Port=19
  VHAL_IVITimeDay_DAY : Outport  Port=20
  VHAL_IVITimeHour_hr : Outport  Port=21
  VHAL_IVITimeMinute_min : Outport  Port=22
  VHAL_IVITimeMonth_MONTH : Outport  Port=23
  VHAL_IVITimeSecond_s : Outport  Port=24
  VHAL_IVITimeYear_YEAR : Outport  Port=25
  VHAL_LINKtoDrive_flg : Outport  Port=26
  VHAL_OpenDrOpenWdoSW_flg : Outport  Port=27
  VHAL_PWCONTINUEUSE_flg : Outport  Port=28
  VHAL_SmartEcoModeSW_flg : Outport  Port=29
  VHAL_UserSet_enum : Outport  Port=30
  wires:
  DT_CAN2_SG_IVI1/1 -> [DT_CAN2_SG_IVI1]
  [DT_CAN2_SG_IVI1] -> bus_selector/1
  bus_selector/1 -> AmbLighLowBatAlertSW/1(AmbLigh_LowBatAlert_SW)  "<CAN2_AmbLigh_LowBatAlert_SW>"
  AmbLighLowBatAlertSW/1(VHAL_AmbLighLowBatAlertSW_flg) -> VHAL_AmbLighLowBatAlertSW_flg/1
  [DT_CAN2_SG_IVI1] -> bus_selector1/1
  bus_selector1/1 -> AmbLighSafetyAlertSW/1(AmbLigh_SafetyAlert_SW)  "<CAN2_AmbLigh_SafetyAlert_SW>"
  AmbLighSafetyAlertSW/1(VHAL_AmbLighSafetyAlertSW_flg) -> VHAL_AmbLighSafetyAlertSW_flg/1
  [DT_CAN2_SG_IVI1] -> bus_selector2/1
  bus_selector2/1 -> AmbLightBrightnessSet/1(AmbLightBrightnessSet)  "<CAN2_AmbLightBrightnessSet>"
  AmbLightBrightnessSet/1(VHAL_AmbLightBrightnessSet_enum) -> VHAL_AmbLightBrightnessSet_enum/1
  [DT_CAN2_SG_IVI1] -> bus_selector3/1
  bus_selector3/1 -> AmbLightColorSet/1(AmbLightColorSet)  "<CAN2_AmbLightColorSet>"
  AmbLightColorSet/1(VHAL_AmbLightColorSet_enum) -> VHAL_AmbLightColorSet_enum/1
  [DT_CAN2_SG_IVI1] -> bus_selector4/1
  bus_selector4/1 -> AmbLightDimInDarkSW/1(AmbLight_DimInDark_SW)  "<CAN2_AmbLight_DimInDark_SW>"
  AmbLightDimInDarkSW/1(VHAL_AmbLightDimInDarkSW_flg) -> VHAL_AmbLightDimInDarkSW_flg/1
  [DT_CAN2_SG_IVI1] -> bus_selector5/1
  bus_selector5/1 -> AmbLightSW/1(AmbLight_SW)  "<CAN2_AmbLight_SW>"
  AmbLightSW/1(VHAL_AmbLightSW_flg) -> VHAL_AmbLightSW_flg/1
  [DT_CAN2_SG_IVI1] -> bus_selector6/1
  bus_selector6/1 -> AmbLightWlcmLightSW/1(AmbLight_WlcmLight_SW)  "<CAN2_AmbLight_WlcmLight_SW>"
  AmbLightWlcmLightSW/1(VHAL_AmbLightWlcmLightSW_flg) -> VHAL_AmbLightWlcmLightSW_flg/1
  [DT_CAN2_SG_IVI1] -> bus_selector7/1
  bus_selector7/1 -> FCPFrEvtBtnACMaxReq/1(FCP_FrEvt_BtnACMaxReq)  "<CAN2_FCP_FrEvt_BtnACMaxReq>"
  FCPFrEvtBtnACMaxReq/1(VHAL_FCPFrEvtBtnACMaxReq_flg) -> VHAL_FCPFrEvtBtnACMaxReq_flg/1
  [DT_CAN2_SG_IVI1] -> bus_selector8/1
  bus_selector8/1 -> FCPFrEvtBtnACReq/1(FCP_FrEvt_BtnACReq)  "<CAN2_FCP_FrEvt_BtnACReq>"
  FCPFrEvtBtnACReq/1(VHAL_FCPFrEvtBtnACReq_flg) -> VHAL_FCPFrEvtBtnACReq_flg/1
  [DT_CAN2_SG_IVI1] -> bus_selector9/1
  bus_selector9/1 -> FCPFrEvtBtnAutoReq/1(FCP_FrEvt_BtnAutoReq)  "<CAN2_FCP_FrEvt_BtnAutoReq>"
  FCPFrEvtBtnAutoReq/1(VHAL_FCPFrEvtBtnAutoReq_flg) -> VHAL_FCPFrEvtBtnAutoReq_flg/1
  [DT_CAN2_SG_IVI1] -> bus_selector10/1
  bus_selector10/1 -> FCPFrEvtBtnSyncReq/1(FCP_FrEvt_BtnSyncReq)  "<CAN2_FCP_FrEvt_BtnSyncReq>"
  FCPFrEvtBtnSyncReq/1(VHAL_FCPFrEvtBtnSyncReq_flg) -> VHAL_FCPFrEvtBtnSyncReq_flg/1
  [DT_CAN2_SG_IVI1] -> bus_selector11/1
  bus_selector11/1 -> IVICreateAccReqSta/1(IVI_CreateAccReq_Sta)  "<CAN2_IVI_CreateAccReq_Sta>"
  IVICreateAccReqSta/1(VHAL_IVICreateAccReqSta_enum) -> VHAL_IVICreateAccReqSta_enum/1
  [DT_CAN2_SG_IVI1] -> bus_selector12/1
  bus_selector12/1 -> IVIDelAccReqSta/1(IVI_DelAccReq_Sta)  "<CAN2_IVI_DelAccReq_Sta>"
  IVIDelAccReqSta/1(VHAL_IVIDelAccReqSta_enum) -> VHAL_IVIDelAccReqSta_enum/1
  [DT_CAN2_SG_IVI1] -> bus_selector13/1
  bus_selector13/1 -> IVILinkAccReqSta/1(IVI_LinkAccReq_Sta)  "<CAN2_IVI_LinkAccReq_Sta>"
  IVILinkAccReqSta/1(VHAL_IVILinkAccReqSta_flg) -> VHAL_IVILinkAccReqSta_flg/1
  [DT_CAN2_SG_IVI1] -> bus_selector14/1
  bus_selector14/1 -> IVILinkAccSta/1(IVI_LinkAcc_Sta)  "<CAN2_IVI_LinkAcc_Sta>"
  IVILinkAccSta/1(VHAL_IVILinkAccSta_enum) -> VHAL_IVILinkAccSta_enum/1
  [DT_CAN2_SG_IVI1] -> bus_selector15/1
  bus_selector15/1 -> IVILinkKeySta/1(IVI_LinkKey_Sta)  "<CAN2_IVI_LinkKey_Sta>"
  IVILinkKeySta/1(VHAL_IVILinkKeySta_enum) -> VHAL_IVILinkKeySta_enum/1
  [DT_CAN2_SG_IVI1] -> bus_selector16/1
  bus_selector16/1 -> IVILocatedSTA/1(IVI_Located_STA)  "<CAN2_IVI_Located_STA>"
  IVILocatedSTA/1(VHAL_IVILocatedSTA_enum) -> VHAL_IVILocatedSTA_enum/1
  [DT_CAN2_SG_IVI1] -> bus_selector17/1
  bus_selector17/1 -> IVILockSoundSWSta/1(IVI_Lock_SoundSW_Sta)  "<CAN2_IVI_Lock_SoundSW_Sta>"
  IVILockSoundSWSta/1(VHAL_IVILockSoundSWSta_flg) -> VHAL_IVILockSoundSWSta_flg/1
  [DT_CAN2_SG_IVI1] -> bus_selector18/1
  bus_selector18/1 -> IVITimeCheck/1(IVI_Time_Check)  "<CAN2_IVI_Time_Check>"
  IVITimeCheck/1(VHAL_IVITimeCheck_enum) -> VHAL_IVITimeCheck_enum/1
  [DT_CAN2_SG_IVI1] -> bus_selector19/1
  bus_selector19/1 -> IVITimeDay/1(IVI_Time_Day)  "<CAN2_IVI_Time_Day>"
  IVITimeDay/1(VHAL_IVITimeDay_DAY) -> VHAL_IVITimeDay_DAY/1
  [DT_CAN2_SG_IVI1] -> bus_selector20/1
  bus_selector20/1 -> IVITimeHour/1(IVI_Time_Hour)  "<CAN2_IVI_Time_Hour>"
  IVITimeHour/1(VHAL_IVITimeHour_hr) -> VHAL_IVITimeHour_hr/1
  [DT_CAN2_SG_IVI1] -> bus_selector21/1
  bus_selector21/1 -> IVITimeMinute/1(IVI_Time_Minute)  "<CAN2_IVI_Time_Minute>"
  IVITimeMinute/1(VHAL_IVITimeMinute_min) -> VHAL_IVITimeMinute_min/1
  [DT_CAN2_SG_IVI1] -> bus_selector22/1
  bus_selector22/1 -> IVITimeMonth/1(IVI_Time_Month)  "<CAN2_IVI_Time_Month>"
  IVITimeMonth/1(VHAL_IVITimeMonth_MONTH) -> VHAL_IVITimeMonth_MONTH/1
  [DT_CAN2_SG_IVI1] -> bus_selector23/1
  bus_selector23/1 -> IVITimeSecond/1(IVI_Time_Second)  "<CAN2_IVI_Time_Second>"
  IVITimeSecond/1(VHAL_IVITimeSecond_s) -> VHAL_IVITimeSecond_s/1
  [DT_CAN2_SG_IVI1] -> bus_selector24/1
  bus_selector24/1 -> IVITimeYear/1(IVI_Time_Year)  "<CAN2_IVI_Time_Year>"
  IVITimeYear/1(VHAL_IVITimeYear_YEAR) -> VHAL_IVITimeYear_YEAR/1
  [DT_CAN2_SG_IVI1] -> bus_selector25/1
  bus_selector25/1 -> LINKtoDrive/1(LINKtoDrive)  "<CAN2_LINKtoDrive>"
  LINKtoDrive/1(VHAL_LINKtoDrive_flg) -> VHAL_LINKtoDrive_flg/1
  [DT_CAN2_SG_IVI1] -> bus_selector26/1
  bus_selector26/1 -> OpenDrOpenWdoSW/1(OpenDrOpenWdo_SW)  "<CAN2_OpenDrOpenWdo_SW>"
  OpenDrOpenWdoSW/1(VHAL_OpenDrOpenWdoSW_flg) -> VHAL_OpenDrOpenWdoSW_flg/1
  [DT_CAN2_SG_IVI1] -> bus_selector27/1
  bus_selector27/1 -> PWCONTINUEUSE/1(PW_CONTINUE_USE)  "<CAN2_PW_CONTINUE_USE>"
  PWCONTINUEUSE/1(VHAL_PWCONTINUEUSE_flg) -> VHAL_PWCONTINUEUSE_flg/1
  [DT_CAN2_SG_IVI1] -> bus_selector28/1
  bus_selector28/1 -> SmartEcoModeSW/1(SmartEco_Mode_SW)  "<CAN2_SmartEco_Mode_SW>"
  SmartEcoModeSW/1(VHAL_SmartEcoModeSW_flg) -> VHAL_SmartEcoModeSW_flg/1
  [DT_CAN2_SG_IVI1] -> bus_selector29/1
  bus_selector29/1 -> UserSet/1(UserSet)  "<CAN2_UserSet>"
  UserSet/1(VHAL_UserSet_enum) -> VHAL_UserSet_enum/1
